simulink model "LCK_old"  (R2018b)
settings: Solver=FixedStepDiscrete  StartTime=0.0  StopTime=inf  FixedStep=0.005  RelTol=1e-3
PostLoadFcn:
  | if any(exist('dsrtsu_mdlpostloadfcn', 'file') ~= 0), dsrtsu_mdlpostloadfcn('Execute', bdroot); end
values from neighbouring files (symbols this model uses):
  C_DEG2RAD = 0.0175    [LCK_Macro.sldd]
  C_KPH2MPS = 0.2778    [LCK_Macro.sldd]
  C_NEARZERO = 0.0001    [LCK_Macro.sldd]
  C_ONE = 1.0    [LCK_Macro.sldd]
  C_RAD2DEG = 57.2958    [LCK_Macro.sldd]
  C_ZERO = 0.0    [LCK_Macro.sldd]
  k_accel_pedal_pos_per_speed_x : value not decoded    [LCK_LogicPara.sldd]
  k_accel_pedal_pos_per_speed_z : value not decoded    [LCK_LogicPara.sldd]
  k_brake_suprress_hold = 1000.0    [LCK_LogicPara.sldd]
  k_driver_appl_torque_filt = 50.0    [LCK_LogicPara.sldd]
  k_driver_suppression_hold_time = 3000.0    [LCK_LogicPara.sldd]
  k_hands_on_wheel_hold_msec = 500.0    [LCK_LogicPara.sldd]
  k_hands_on_wheel_torque_hi = 0.2    [LCK_LogicPara.sldd]
  k_hands_on_wheel_torque_lo = 0.15    [LCK_LogicPara.sldd]
  k_handsoff_delay_cycles = 50.0    [LCK_LogicPara.sldd]
  k_handsoff_torq_Lo_CR = 0.3    [LCK_LogicPara.sldd]
  k_handson_delay_cycles = 5.0    [LCK_LogicPara.sldd]
  k_HighAccel_suppress_hold = 3000.0    [LCK_LogicPara.sldd]
  k_HLR_suprress_hold = 3000.0    [LCK_LogicPara.sldd]
  k_hs_StrAng_CR_threshold_z : value not decoded    [LCK_LogicPara.sldd]
  k_LC_Exit_Switch = 0.0    [LCK_LogicPara.sldd]
  k_LCG_Configured = 1.0    [LCK_LogicPara.sldd]
  k_LCK_A0_Rdy2Act_UseConst = 0.0    [LCK_LogicPara.sldd]
  k_LCK_A0Fac_ActSta : value not decoded    [LCK_CtrlPara.sldd]
  k_LCK_A0Fac_DrvStm : value not decoded    [LCK_CtrlPara.sldd]
  k_LCK_A0Shift_LftCurv : value not decoded    [LCK_CtrlPara.sldd]
  k_LCK_A0Shift_RgtCurv : value not decoded    [LCK_CtrlPara.sldd]
  k_LCK_A0Shift_StraLan = 0.0    [LCK_CtrlPara.sldd]
  k_LCK_A0ShiftFac_Dy_LftCurv : value not decoded    [LCK_CtrlPara.sldd]
  k_LCK_A0ShiftFac_Dy_RgtCurv : value not decoded    [LCK_CtrlPara.sldd]
  k_LCK_A0ShiftFac_Vspd : value not decoded    [LCK_CtrlPara.sldd]
  k_LCK_accel_inhibit_thold = 35.0    [LCK_LogicPara.sldd]
  k_LCK_Active2Ready_Mask = 255.0    [LCK_LogicPara.sldd]
  k_LCK_CvatRateBks : value not decoded    [LCK_CtrlPara.sldd]
  k_LCK_CvatrBks : value not decoded    [LCK_CtrlPara.sldd]
  k_LCK_DFac_Dy : value not decoded    [LCK_CtrlPara.sldd]
  k_LCK_DFac_Dy_Curv : value not decoded    [LCK_CtrlPara.sldd]
  k_LCK_DFac_HaCurCen : value not decoded    [LCK_CtrlPara.sldd]
  k_LCK_DFac_HaCurSid : value not decoded    [LCK_CtrlPara.sldd]
  k_LCK_DFac_HadCurCen : value not decoded    [LCK_CtrlPara.sldd]
  k_LCK_DFac_HadCurSid : value not decoded    [LCK_CtrlPara.sldd]
  k_LCK_DFac_HadStrCen : value not decoded    [LCK_CtrlPara.sldd]
  k_LCK_DFac_HadStrSid : value not decoded    [LCK_CtrlPara.sldd]
  k_LCK_DFac_HaStrCen : value not decoded    [LCK_CtrlPara.sldd]
  k_LCK_DFac_HaStrSid : value not decoded    [LCK_CtrlPara.sldd]
  k_LCK_DFac_Rad : value not decoded    [LCK_CtrlPara.sldd]
  k_LCK_DFac_SA_CurCen : value not decoded    [LCK_CtrlPara.sldd]
  k_LCK_DFac_SA_CurSid : value not decoded    [LCK_CtrlPara.sldd]
  k_LCK_DFac_SA_StrCen : value not decoded    [LCK_CtrlPara.sldd]
  k_LCK_DFac_SA_StrSid : value not decoded    [LCK_CtrlPara.sldd]
  k_LCK_DFac_SS_CurCen : value not decoded    [LCK_CtrlPara.sldd]
  k_LCK_DFac_SS_CurSid : value not decoded    [LCK_CtrlPara.sldd]
  k_LCK_DFac_SS_StrCen : value not decoded    [LCK_CtrlPara.sldd]
  k_LCK_DFac_SS_StrSid : value not decoded    [LCK_CtrlPara.sldd]
  k_LCK_DFac_Vspd : value not decoded    [LCK_CtrlPara.sldd]
  k_LCK_DlyTm_DrvStim = 0.2    [LCK_CtrlPara.sldd]
  k_LCK_DTermMax = 2.0    [LCK_CtrlPara.sldd]
  k_LCK_DyBks_Curv : value not decoded    [LCK_CtrlPara.sldd]
  k_LCK_Enable_POOnly = 1.0    [LCK_LogicPara.sldd]
  k_LCK_Entry_DistBuffer = 0.1    [LCK_LogicPara.sldd]
  k_LCK_Fac_Vspd2RngThr_FalRec = 0.23    [LCK_CtrlPara.sldd]
  k_LCK_Ffw_CvatSwh = 0.0    [LCK_CtrlPara.sldd]
  k_LCK_Ffw_DyBks : value not decoded    [LCK_CtrlPara.sldd]
  k_LCK_Ffw_TimCon_CmdFlt = 0.0    [LCK_CtrlPara.sldd]
  k_LCK_FfwDeltaFac_Rad_Lft : value not decoded    [LCK_CtrlPara.sldd]
  k_LCK_FfwDeltaFac_Rad_Rgt : value not decoded    [LCK_CtrlPara.sldd]
  k_LCK_FfwDeltaFac_Vspd : value not decoded    [LCK_CtrlPara.sldd]
  k_LCK_FfwFac_CvatRate_Lft : value not decoded    [LCK_CtrlPara.sldd]
  k_LCK_FfwFac_CvatRate_Rgt : value not decoded    [LCK_CtrlPara.sldd]
  k_LCK_FfwFac_Dy : value not decoded    [LCK_CtrlPara.sldd]
  k_LCK_FfwFac_Rad_Lft : value not decoded    [LCK_CtrlPara.sldd]
  k_LCK_FfwFac_Rad_Rgt : value not decoded    [LCK_CtrlPara.sldd]
  k_LCK_FfwFac_Vspd : value not decoded    [LCK_CtrlPara.sldd]
  k_LCK_FfwTorq_Cvat : value not decoded    [LCK_CtrlPara.sldd]
  k_LCK_HAFac_ActSta : value not decoded    [LCK_CtrlPara.sldd]
  k_LCK_HAFac_DrvStm : value not decoded    [LCK_CtrlPara.sldd]
  k_LCK_HaloTime = 2000.0    [LCK_LogicPara.sldd]
  k_LCK_HaloTime_Switch = 0.0    [LCK_LogicPara.sldd]
  k_LCK_HARFac_ActSta : value not decoded    [LCK_CtrlPara.sldd]
  k_LCK_HARFac_DrvStm : value not decoded    [LCK_CtrlPara.sldd]
  k_LCK_Hed_DyBks : value not decoded    [LCK_CtrlPara.sldd]
  k_LCK_HedAngDiffX : value not decoded    [LCK_CtrlPara.sldd]
  k_LCK_HedAngRateDiffX : value not decoded    [LCK_CtrlPara.sldd]
  k_LCK_HndsOnWhel_DlyTm_Idl2Rdy = 0.0    [LCK_LogicPara.sldd]
  k_LCK_host_veh_width = 1.86    [LCK_LogicPara.sldd]
  k_LCK_Idle2Ready_Mask = 239.0    [LCK_LogicPara.sldd]
  k_LCK_Junc_SusTime = 1.0    [LCK_LogicPara.sldd]
  k_LCK_KpKdDecSlopeLmt = 10.0    [LCK_CtrlPara.sldd]
  k_LCK_KpKdIncSlopeLmt = 5.0    [LCK_CtrlPara.sldd]
  k_LCK_Lat_Ctrl_DFac_Lft = 1.0    [LCK_CtrlPara.sldd]
  k_LCK_Lat_Ctrl_DFac_Rgt = 1.05    [LCK_CtrlPara.sldd]
  k_LCK_Lat_Ctrl_Kd = 0.8    [LCK_CtrlPara.sldd]
  k_LCK_Lat_Ctrl_Ki = 0.5    [LCK_CtrlPara.sldd]
  k_LCK_Lat_Ctrl_Kp = 0.7    [LCK_CtrlPara.sldd]
  k_LCK_Lat_Ctrl_Kp_NearGain = 0.7    [LCK_CtrlPara.sldd]
  k_LCK_Lat_Ctrl_PFac_Lft = 1.0    [LCK_CtrlPara.sldd]
  k_LCK_Lat_Ctrl_PFac_Rgt = 1.05    [LCK_CtrlPara.sldd]
  k_LCK_Lat_Ctrl_TimCon_CmdFlt = 5.0    [LCK_CtrlPara.sldd]
  k_LCK_Lat_DFac_Rad : value not decoded    [LCK_CtrlPara.sldd]
  k_LCK_Lat_DFac_SS_Cur : value not decoded    [LCK_CtrlPara.sldd]
  k_LCK_Lat_DFac_SS_Str : value not decoded    [LCK_CtrlPara.sldd]
  k_LCK_Lat_DFac_Vspd : value not decoded    [LCK_CtrlPara.sldd]
  k_LCK_Lat_DyBks : value not decoded    [LCK_CtrlPara.sldd]
  k_LCK_Lat_IFac_Rad : value not decoded    [LCK_CtrlPara.sldd]
  k_LCK_Lat_IFac_Vspd : value not decoded    [LCK_CtrlPara.sldd]
  k_LCK_Lat_ILmtFac_Dy_CurvLan : value not decoded    [LCK_CtrlPara.sldd]
  k_LCK_Lat_ILmtFac_Dy_StraLan : value not decoded    [LCK_CtrlPara.sldd]
  k_LCK_Lat_ILmtFac_Rad : value not decoded    [LCK_CtrlPara.sldd]
  k_LCK_Lat_ILmtFac_Rad_NearGain = 1.0    [LCK_CtrlPara.sldd]
  k_LCK_Lat_ILmtFac_Vspd_CurvLan : value not decoded    [LCK_CtrlPara.sldd]
  k_LCK_Lat_ILmtFac_Vspd_StraLan : value not decoded    [LCK_CtrlPara.sldd]
  k_LCK_Lat_ITermLmt_Dy = 1.0    [LCK_CtrlPara.sldd]
  k_LCK_Lat_KpKdDecSlopeLmt = 10.0    [LCK_CtrlPara.sldd]
  k_LCK_Lat_KpKdIncSlopeLmt = 10.0    [LCK_CtrlPara.sldd]
  k_LCK_Lat_PFac_Dy_InnLftCur : value not decoded    [LCK_CtrlPara.sldd]
  k_LCK_Lat_PFac_Dy_InnRgtCur : value not decoded    [LCK_CtrlPara.sldd]
  k_LCK_Lat_PFac_Dy_OutLftCur : value not decoded    [LCK_CtrlPara.sldd]
  k_LCK_Lat_PFac_Dy_OutRgtCur : value not decoded    [LCK_CtrlPara.sldd]
  k_LCK_Lat_PFac_Dy_Str : value not decoded    [LCK_CtrlPara.sldd]
  k_LCK_Lat_PFac_Rad : value not decoded    [LCK_CtrlPara.sldd]
  ... (+158 more)
undefined symbols (not defined in the file or in its folder): k_LCK_CurvBks, K_LCK_SPA0A1A2_LMRngCmp_y
libraries: LateralControl_fcns_lib x58, simulink x22
(part 4 of 45)

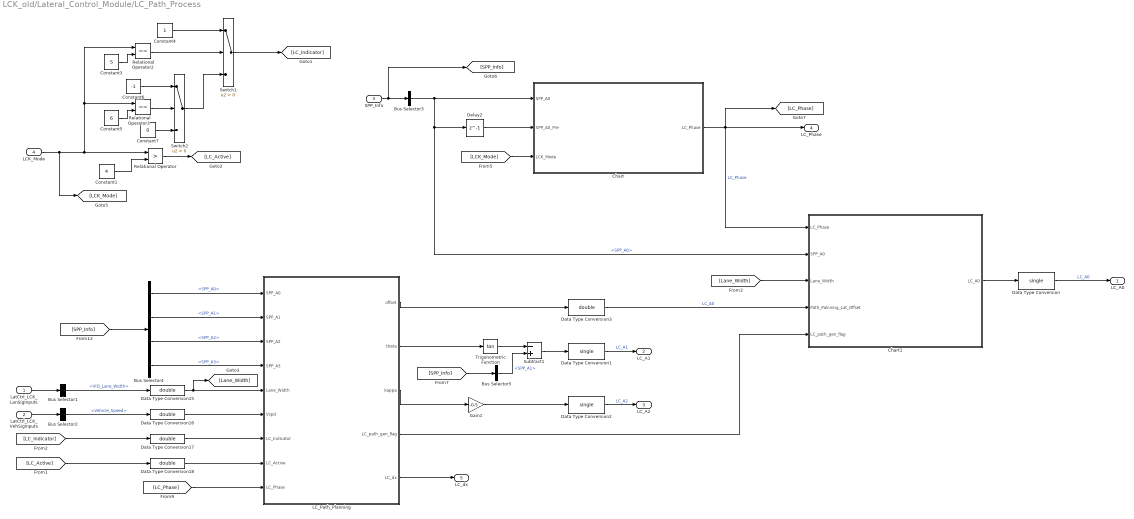
== system LCK_old/Lateral_Control_Module/LC_Path_Process ==
  LatCtrl_LCK_LanSigInputs : Inport  OutDataTypeStr=Bus: LatCtrl_LCK_LanSigInputs_t
  LatCtrl_LCK_VehSigInputs : Inport  Description=_GWMAB30P4.LCK.000_287_  Port=2  OutDataTypeStr=Bus: LatCtrl_LCK_VehSigInputs_t
  SPP_Info : Inport  Port=3
  LCK_Mode : Inport  Port=4
  Bus Selector1 : BusSelector  OutputSignals=VID_Lane_Width
  Bus Selector2 : BusSelector  OutputSignals=Vehicle_Speed
  Bus Selector3 : BusSelector  OutputSignals=SPP_A0
  Bus Selector4 : BusSelector  OutputSignals=SPP_A0,SPP_A1,SPP_A2,SPP_A3
  Bus Selector5 : BusSelector  OutputSignals=SPP_A1
  Chart : Stateflow chart  TreatAsAtomicUnit=on
  Chart1 : Stateflow chart  TreatAsAtomicUnit=on
  Constant1 : Constant  Value=4
  Constant3 : Constant  Value=5
  Constant4 : Constant
  Constant5 : Constant  Value=6
  Constant6 : Constant  Value=-1
  Constant7 : Constant  Value=0
  Data Type Conversion : DataTypeConversion  OutDataTypeStr=single
  Data Type Conversion1 : DataTypeConversion  OutDataTypeStr=single
  Data Type Conversion{3,15..18} (5 alike) : DataTypeConversion  OutDataTypeStr=double
  Data Type Conversion2 : DataTypeConversion  OutDataTypeStr=single
  Delay2 : Delay  DelayLength=1  InitialCondition=0
  Gain1 : Gain  Gain=-0.5
  LC_Path_Planning : Subsystem
  Relational Operator : RelationalOperator  Operator=>  OutDataTypeStr=boolean  RndMeth=Simplest
  Relational Operator2 : RelationalOperator  Operator===  OutDataTypeStr=boolean  RndMeth=Simplest
  Relational Operator3 : RelationalOperator  Operator===  OutDataTypeStr=boolean  RndMeth=Simplest
  Subtract1 : Sum  Inputs=-+
  Switch1 : Switch  Criteria=u2 > Threshold
  Switch2 : Switch  Criteria=u2 > Threshold
  Trigonometric Function : Trigonometry  Operator=tan
  LC_A0 : Outport  Description=_GWMAB30P4.LCK.000_194_
  LC_A1 : Outport  Description=_GWMAB30P4.LCK.000_194_  Port=2
  LC_A2 : Outport  Description=_GWMAB30P4.LCK.000_194_  Port=3
  LC_Phase : Outport  Description=_GWMAB30P4.LCK.000_194_  Port=4
  LC_dx : Outport  Port=5
  wires:
  Relational Operator/1 -> [LC_Active]
  LCK_Mode/1 -> [LCK_Mode], Relational Operator2/1, Relational Operator3/1, Relational Operator/1
  Constant1/1 -> Relational Operator/2
  LatCtrl_LCK_LanSigInputs/1 -> Bus Selector1/1
  [LC_Active] -> Data Type Conversion18/1
  Constant3/1 -> Relational Operator2/2
  Relational Operator2/1 -> Switch1/2
  Constant4/1 -> Switch1/1
  Constant5/1 -> Relational Operator3/2
  Relational Operator3/1 -> Switch2/2
  Constant6/1 -> Switch2/1
  Switch2/1 -> Switch1/3
  Constant7/1 -> Switch2/3
  Switch1/1 -> [LC_Indicator]
  [LC_Indicator] -> Data Type Conversion17/1
  LatCtrl_LCK_VehSigInputs/1 -> Bus Selector2/1
  Bus Selector2/1 -> Data Type Conversion16/1  "<Vehicle_Speed>"
  SPP_Info/1 -> [SPP_Info], Bus Selector3/1
  Bus Selector3/1 -> Chart1/2(SPP_A0), Delay2/1, Chart/1(SPP_A0)  "<SPP_A0>"
  Delay2/1 -> Chart/2(SPP_A0_Pre)
  [LCK_Mode] -> Chart/3(LCK_Mode)
  Bus Selector1/1 -> Data Type Conversion15/1  "<VID_Lane_Width>"
  Data Type Conversion/1 -> LC_A0/1  "LC_A0"
  Data Type Conversion1/1 -> LC_A1/1  "LC_A1"
  Data Type Conversion2/1 -> LC_A2/1  "LC_A2"
  Data Type Conversion15/1 -> [Lane_Width], LC_Path_Planning/5(Lane_Width)
  Data Type Conversion16/1 -> LC_Path_Planning/6(Vspd)
  Data Type Conversion17/1 -> LC_Path_Planning/7(LC_Indicator)
  Data Type Conversion18/1 -> LC_Path_Planning/8(LC_Active)
  Chart/1(LC_Phase) -> Chart1/1(LC_Phase), LC_Phase/1, [LC_Phase]  "LC_Phase"
  [SPP_Info] -> Bus Selector5/1
  Bus Selector5/1 -> Subtract1/2  "<SPP_A1>"
  Trigonometric Function/1 -> Subtract1/1
  Subtract1/1 -> Data Type Conversion1/1
  LC_Path_Planning/2(theta) -> Trigonometric Function/1
  [LC_Phase] -> LC_Path_Planning/9(LC_Phase)
  [SPP_Info] -> Bus Selector4/1
  Bus Selector4/1 -> LC_Path_Planning/1(SPP_A0)  "<SPP_A0>"
  Bus Selector4/2 -> LC_Path_Planning/2(SPP_A1)  "<SPP_A1>"
  Bus Selector4/3 -> LC_Path_Planning/3(SPP_A2)  "<SPP_A2>"
  Bus Selector4/4 -> LC_Path_Planning/4(SPP_A3)  "<SPP_A3>"
  LC_Path_Planning/3(kappa) -> Gain1/1
  Gain1/1 -> Data Type Conversion2/1
  LC_Path_Planning/1(offset) -> Data Type Conversion3/1
  Chart1/1(LC_A0) -> Data Type Conversion/1
  [Lane_Width] -> Chart1/3(Lane_Width)
  Data Type Conversion3/1 -> Chart1/4(Path_Palnning_Lat_Offset)  "LC_A0"
  LC_Path_Planning/4(LC_path_gen_flag) -> Chart1/5(LC_path_gen_flag)
  LC_Path_Planning/5(LC_dx) -> LC_dx/1

== system LCK_old/Lateral_Control_Module/Lat_HMI ==
  Driver_Operation_Info : Inport  Description=_GWMH9P3.Latctrl.000_23_
  LCK_Mode : Inport  Description=_GWMH9P3.Latctrl.000_23_  Port=2
  LC_dx : Inport  Description=_GWMH9P3.Latctrl.000_23_  Port=3
  Bus Creator : BusCreator  Inputs=13  OutDataTypeStr=Bus: HMI_Lateral_t
      settings: InheritFromInputs=off
  Bus Selector : BusSelector  OutputSignals=f_hands_on_wheel
  Constant1 : Constant  Value=4
  Constant2 : Constant  Value=0  OutDataTypeStr=single
  Constant29 : Constant  Value=0
  Constant3 : Constant  Value=5
  Constant4 : Constant
  Constant5 : Constant  Value=6
  Constant6 : Constant  Value=2
  Constant7 : Constant  Value=0
  Data Type Conversion{,1..3} (4 alike) : DataTypeConversion  OutDataTypeStr=single
  Logical Operator : Logic  Operator=NOT  AllPortsSameDT=off  OutDataTypeStr=boolean
  Relational Operator{1..3,20} (4 alike) : RelationalOperator  Operator===  OutDataTypeStr=boolean  RndMeth=Simplest
  Switch1 : Switch  Criteria=u2 > Threshold
  Switch2 : Switch  Criteria=u2 > Threshold
  Lateral_HMI : Outport  Description=_GWMAB30P4.LCK.000_194_  OutDataTypeStr=Bus: HMI_Lateral_t
  wires:
  Bus Creator/1 -> Lateral_HMI/1
  Constant29/1 -> Relational Operator20/2
  Relational Operator20/1 -> Data Type Conversion/1
  Constant1/1 -> Relational Operator1/2
  Relational Operator1/1 -> Data Type Conversion1/1
  Constant2/1 -> Bus Creator/6, Bus Creator/7, Bus Creator/8, Bus Creator/9, Bus Creator/10, Bus Creator/5, Bus Creator/4
  Driver_Operation_Info/1 -> Bus Selector/1
  Bus Selector/1 -> Logical Operator/1  "<f_hands_on_wheel>"
  Data Type Conversion/1 -> Bus Creator/1
  Data Type Conversion1/1 -> Bus Creator/2
  Logical Operator/1 -> Data Type Conversion2/1
  Data Type Conversion2/1 -> Bus Creator/13
  Constant6/1 -> Switch2/1
  Switch2/1 -> Switch1/3
  Constant7/1 -> Switch2/3
  LCK_Mode/1 -> Relational Operator20/1, Relational Operator1/1, Bus Creator/3, Relational Operator2/1, Relational Operator3/1
  Relational Operator3/1 -> Switch2/2
  Relational Operator2/1 -> Switch1/2
  Constant4/1 -> Switch1/1
  Constant3/1 -> Relational Operator2/2
  Constant5/1 -> Relational Operator3/2
  Switch1/1 -> Data Type Conversion3/1
  LC_dx/1 -> Bus Creator/11
  Data Type Conversion3/1 -> Bus Creator/12
